simulink model "validation_model"  (R2018b)
settings: Solver=VariableStepAuto  StartTime=0.0  StopTime=10.0  RelTol=1e-3
values from neighbouring files (symbols this model uses):
  A_bike = [0 g/h_real ; 1 0]    [configuration.m]
  B_bike = [1 ; 0]    [configuration.m]
  C1_bike = a_real/(b_real*h_real)    (= 0.392543973584)    [configuration.m]
  C2_bike = 1/(b_real*h_real)    (= 1.15454109878)    [configuration.m]
  C_ini = [C1_bike*input_velocity C2_bike*input_velocity^2]    [configuration.m]
  D = zeros(3,1)    [configuration_pidTuning.m]
  delay_tf_steering = 0    [configuration.m]
  initial_states = [deg2rad(-2) deg2rad(0) deg2rad(0)]    [configuration.m]    (also in configuration_pidTuning.m)
  K_fullbike = 1    [configuration.m]
  lqr_gains = zeros(length(velocity_lqr),1+size(A_bike,1))    [lqr_design.m]
  smith_fullbike = 1    [configuration.m]
  Ts = 0.01    [configuration.m]    (also in configuration_pidTuning.m = 0.04)
  velocity_lqr = [input_velocity - 0.1 , input_velocity , input_velocity + 0.1]    [lqr_design.m]
settings Model: Creator=maximef  LastModifiedBy=maximef

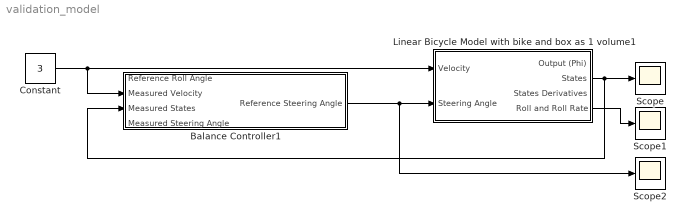
== system validation_model ==
  Balance Controller1 : Subsystem  SystemSampleTime=Ts
  Constant : Constant  Value=3
  Linear Bicycle Model with bike and box as 1 volume1 : Subsystem
  Scope : Scope
  Scope1 : Scope
  Scope2 : Scope
  wires:
  Balance Controller1/1(Reference Steering Angle) -> Scope2/1, Linear Bicycle Model with bike and box as 1 volume1/2(Steering Angle)
  Constant/1 -> Balance Controller1/2(Measured Velocity), Linear Bicycle Model with bike and box as 1 volume1/1(Velocity)
  Linear Bicycle Model with bike and box as 1 volume1/2(States) -> Scope/1, Balance Controller1/3(Measured States)
  Linear Bicycle Model with bike and box as 1 volume1/4(Roll and Roll Rate) -> Scope1/1

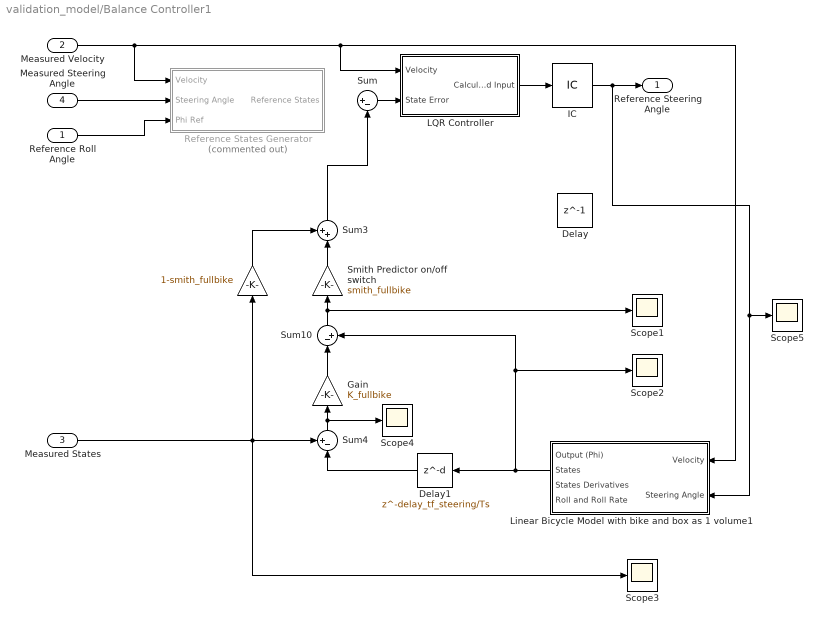
== system validation_model/Balance Controller1 ==
  Reference Roll Angle : Inport
  Measured Velocity : Inport  Port=2
  Measured States : Inport  Port=3
  Measured Steering Angle : Inport  Port=4
  " " : Gain  Gain=1-smith_fullbike
  Delay : Delay  DelayLength=1
  Delay1 : Delay  DelayLength=delay_tf_steering/Ts  SampleTime=Ts
  Gain : Gain  Gain=K_fullbike
  IC : InitialCondition  Value=0
  LQR Controller : Subsystem  TreatAsAtomicUnit=on  SystemSampleTime=Ts
  Linear Bicycle Model with bike and box as 1 volume1 : Subsystem
  Reference States Generator : Subsystem  Commented=on  SystemSampleTime=Ts
  Scope{1..5} (5 alike) : Scope
  Smith Predictor on/off switch : Gain  Gain=smith_fullbike
  Sum : Sum  Inputs=|+-
  Sum10 : Sum  Inputs=|-+
  Sum3 : Sum  Inputs=++|
  Sum4 : Sum  Inputs=+-|
  Reference Steering Angle : Outport
  wires:
  Sum/1 -> LQR Controller/2(State Error)
  LQR Controller/1(Calculated Input) -> IC/1
  Measured Velocity/1 -> Linear Bicycle Model with bike and box as 1 volume1/1(Velocity), LQR Controller/1(Velocity), Reference States Generator/1(Velocity)
  Reference Roll Angle/1 -> Reference States Generator/3(Phi Ref)
  Measured Steering Angle/1 -> Reference States Generator/2(Steering Angle)
  Measured States/1 -> " "/1, Scope3/1, Sum4/1
  " "/1 -> Sum3/1
  Sum3/1 -> Sum/2
  Linear Bicycle Model with bike and box as 1 volume1/2(States) -> Sum10/2, Scope2/1, Delay1/1
  Gain/1 -> Sum10/1
  Delay1/1 -> Sum4/2
  Smith Predictor on/off switch/1 -> Sum3/2
  Sum10/1 -> Scope1/1, Smith Predictor on/off switch/1
  Sum4/1 -> Scope4/1, Gain/1
  IC/1 -> Linear Bicycle Model with bike and box as 1 volume1/2(Steering Angle), Scope5/1, Reference Steering Angle/1

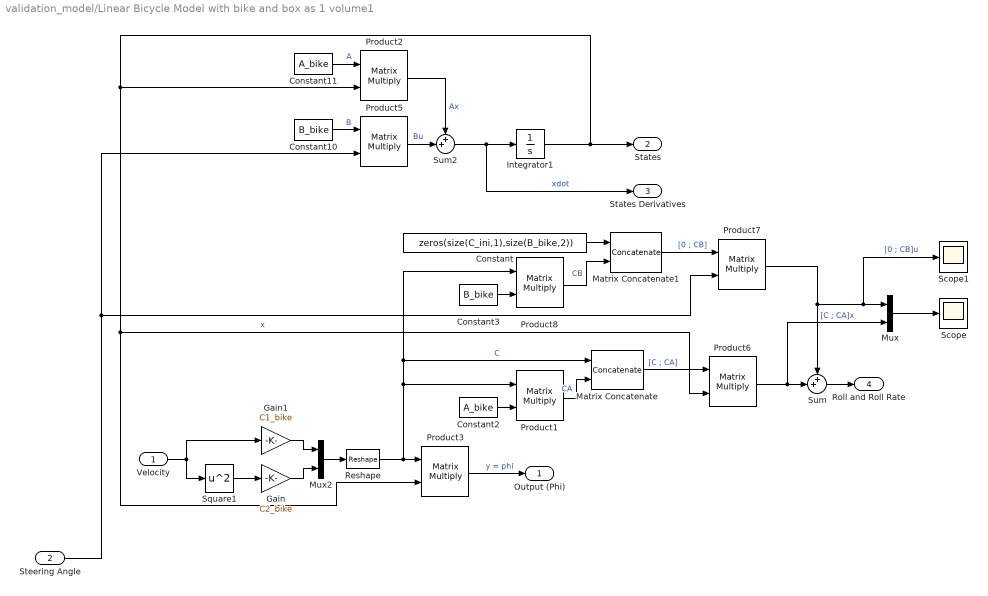
== system validation_model/Linear Bicycle Model with bike and box as 1 volume1 ==
  Velocity : Inport
  Steering Angle : Inport  Port=2
  Constant : Constant  Value=zeros(size(C_ini,1),size(B_bike,2))
  Constant10 : Constant  Value=B_bike
  Constant11 : Constant  Value=A_bike
  Constant2 : Constant  Value=A_bike
  Constant3 : Constant  Value=B_bike
  Gain : Gain  Gain=C2_bike
  Gain1 : Gain  Gain=C1_bike
  Integrator1 : Integrator  InitialCondition=[C_ini ; C_ini*A_bike]\[initial_states(1) ; initial_states(3)]
  Matrix Concatenate : Concatenate  Mode=Multidimensional array
  Matrix Concatenate1 : Concatenate  Mode=Multidimensional array
  Mux : Mux  Inputs=2
  Mux2 : Mux  Inputs=2
  Product{1..3,5..8} (7 alike) : Product  SCDEnableBlockLinearizationSpecification=on  Multiplication=Matrix(*)
  Reshape : Reshape  OutputDimensionality=Row vector (2-D)
  Scope : Scope
  Scope1 : Scope
  Square1 : Math  Operator=square  SaturateOnIntegerOverflow=on
  Sum : Sum  Inputs=++|
  Sum2 : Sum  Inputs=++|
  Output (Phi) : Outport
  States : Outport  Port=2
  States Derivatives : Outport  Port=3
  Roll and Roll Rate : Outport  Port=4
  wires:
  Integrator1/1 -> Product2/2, Product6/2, Product3/2, States/1  "x"
  Product3/1 -> Output (Phi)/1  "y = phi"
  Steering Angle/1 -> Product5/2, Product7/2
  Product2/1 -> Sum2/1  "Ax"
  Mux2/1 -> Reshape/1
  Product5/1 -> Sum2/2  "Bu"
  Sum2/1 -> Integrator1/1, States Derivatives/1  "xdot"
  Constant11/1 -> Product2/1  "A"
  Constant10/1 -> Product5/1  "B"
  Velocity/1 -> Gain1/1, Square1/1
  Square1/1 -> Gain/1
  Reshape/1 -> Product3/1, Product8/1, Matrix Concatenate/1, Product1/1  "C"
  Gain/1 -> Mux2/2
  Gain1/1 -> Mux2/1
  Sum/1 -> Roll and Roll Rate/1
  Constant2/1 -> Product1/2
  Product1/1 -> Matrix Concatenate/2  "CA"
  Matrix Concatenate/1 -> Product6/1  "[C ; CA]"
  Product6/1 -> Mux/2, Sum/2  "[C ; CA]x"
  Product7/1 -> Scope1/1, Mux/1, Sum/1  "[0 ; CB]u"
  Matrix Concatenate1/1 -> Product7/1  "[0 ; CB]"
  Product8/1 -> Matrix Concatenate1/2  "CB"
  Constant3/1 -> Product8/2
  Constant/1 -> Matrix Concatenate1/1
  Mux/1 -> Scope/1

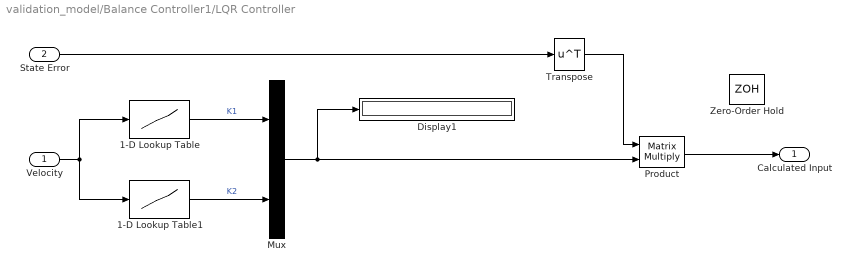
== system validation_model/Balance Controller1/LQR Controller ==
  Velocity : Inport
  State Error : Inport  Port=2
  1-D Lookup Table : Lookup_n-D  NumberOfTableDimensions=1  BreakpointsForDimension1=velocity_lqr  BreakpointsForDimension2=velocity_lqr  BreakpointsForDimension3=velocity_lqr  BreakpointsForDimension4=velocity_lqr  Table=lqr_gains(:,2)  InternalRulePriority=Speed  RndMeth=Simplest  InputSameDT=on
  1-D Lookup Table1 : Lookup_n-D  NumberOfTableDimensions=1  BreakpointsForDimension1=velocity_lqr  BreakpointsForDimension2=velocity_lqr  BreakpointsForDimension3=velocity_lqr  BreakpointsForDimension4=velocity_lqr  Table=lqr_gains(:,3)  InternalRulePriority=Speed  RndMeth=Simplest  InputSameDT=on
  Display1 : Display
  Mux : Mux  Inputs=2
  Product : Product  Multiplication=Matrix(*)
  Transpose : Math  Operator=transpose  SaturateOnIntegerOverflow=on
  Zero-Order Hold : ZeroOrderHold  SampleTime=Ts
  Calculated Input : Outport
  wires:
  1-D Lookup Table/1 -> Mux/1  "K1"
  1-D Lookup Table1/1 -> Mux/2  "K2"
  Velocity/1 -> 1-D Lookup Table1/1, 1-D Lookup Table/1
  Mux/1 -> Product/2, Display1/1
  Transpose/1 -> Product/1
  Product/1 -> Calculated Input/1
  State Error/1 -> Transpose/1

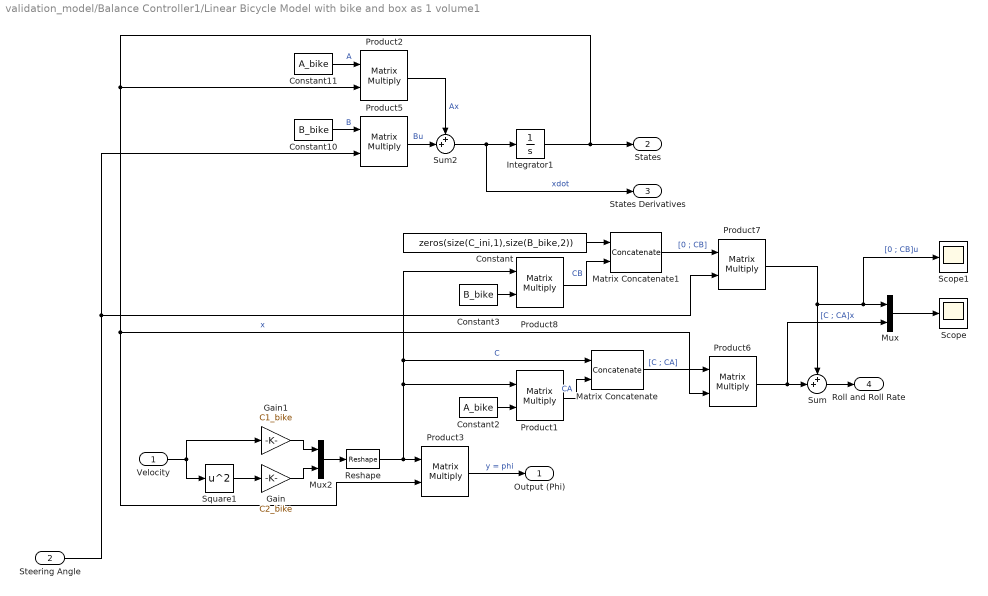
== system validation_model/Balance Controller1/Linear Bicycle Model with bike and box as 1 volume1 ==
  Velocity : Inport
  Steering Angle : Inport  Port=2
  Constant : Constant  Value=zeros(size(C_ini,1),size(B_bike,2))
  Constant10 : Constant  Value=B_bike
  Constant11 : Constant  Value=A_bike
  Constant2 : Constant  Value=A_bike
  Constant3 : Constant  Value=B_bike
  Gain : Gain  Gain=C2_bike
  Gain1 : Gain  Gain=C1_bike
  Integrator1 : Integrator  InitialCondition=[C_ini ; C_ini*A_bike]\[initial_states(1) ; initial_states(3)]
  Matrix Concatenate : Concatenate  Mode=Multidimensional array
  Matrix Concatenate1 : Concatenate  Mode=Multidimensional array
  Mux : Mux  Inputs=2
  Mux2 : Mux  Inputs=2
  Product{1..3,5..8} (7 alike) : Product  SCDEnableBlockLinearizationSpecification=on  Multiplication=Matrix(*)
  Reshape : Reshape  OutputDimensionality=Row vector (2-D)
  Scope : Scope
  Scope1 : Scope
  Square1 : Math  Operator=square  SaturateOnIntegerOverflow=on
  Sum : Sum  Inputs=++|
  Sum2 : Sum  Inputs=++|
  Output (Phi) : Outport
  States : Outport  Port=2
  States Derivatives : Outport  Port=3
  Roll and Roll Rate : Outport  Port=4
  wires:
  Integrator1/1 -> Product2/2, Product6/2, Product3/2, States/1  "x"
  Product3/1 -> Output (Phi)/1  "y = phi"
  Steering Angle/1 -> Product5/2, Product7/2
  Product2/1 -> Sum2/1  "Ax"
  Mux2/1 -> Reshape/1
  Product5/1 -> Sum2/2  "Bu"
  Sum2/1 -> Integrator1/1, States Derivatives/1  "xdot"
  Constant11/1 -> Product2/1  "A"
  Constant10/1 -> Product5/1  "B"
  Velocity/1 -> Gain1/1, Square1/1
  Square1/1 -> Gain/1
  Reshape/1 -> Product3/1, Product8/1, Matrix Concatenate/1, Product1/1  "C"
  Gain/1 -> Mux2/2
  Gain1/1 -> Mux2/1
  Sum/1 -> Roll and Roll Rate/1
  Constant2/1 -> Product1/2
  Product1/1 -> Matrix Concatenate/2  "CA"
  Matrix Concatenate/1 -> Product6/1  "[C ; CA]"
  Product6/1 -> Mux/2, Sum/2  "[C ; CA]x"
  Product7/1 -> Scope1/1, Mux/1, Sum/1  "[0 ; CB]u"
  Matrix Concatenate1/1 -> Product7/1  "[0 ; CB]"
  Product8/1 -> Matrix Concatenate1/2  "CB"
  Constant3/1 -> Product8/2
  Constant/1 -> Matrix Concatenate1/1
  Mux/1 -> Scope/1

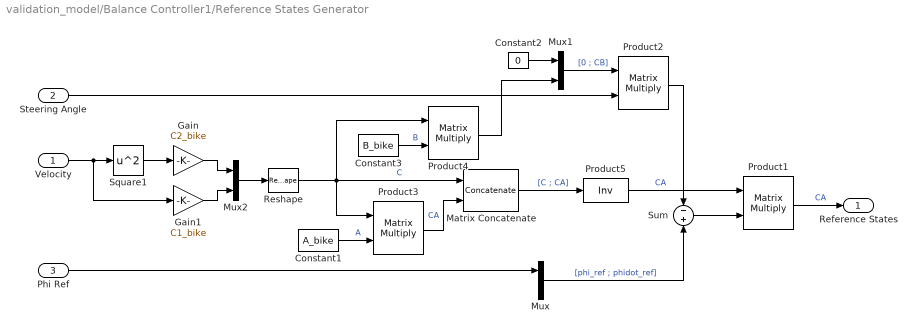
== system validation_model/Balance Controller1/Reference States Generator ==
  Velocity : Inport
  Steering Angle : Inport  Port=2
  Phi Ref : Inport  Port=3
  Constant1 : Constant  Value=A_bike
  Constant2 : Constant  Value=0
  Constant3 : Constant  Value=B_bike
  Gain : Gain  Gain=C2_bike
  Gain1 : Gain  Gain=C1_bike
  Matrix Concatenate : Concatenate  Mode=Multidimensional array
  Mux : Mux  Inputs=2
  Mux1 : Mux  Inputs=2
  Mux2 : Mux  Inputs=2
  Product{1..4} (4 alike) : Product  SCDEnableBlockLinearizationSpecification=on  Multiplication=Matrix(*)
  Product5 : Product  SCDEnableBlockLinearizationSpecification=on  Inputs=/  Multiplication=Matrix(*)
  Reshape : Reshape  OutputDimensionality=Row vector (2-D)
  Square1 : Math  Operator=square  SaturateOnIntegerOverflow=on
  Sum : Sum  Inputs=-+
  Reference States : Outport
  wires:
  Velocity/1 -> Gain1/1, Square1/1
  Gain1/1 -> Mux2/2
  Gain/1 -> Mux2/1
  Square1/1 -> Gain/1
  Reshape/1 -> Product4/1, Matrix Concatenate/1, Product3/1  "C"
  Mux2/1 -> Reshape/1
  Constant1/1 -> Product3/2  "A"
  Product3/1 -> Matrix Concatenate/2  "CA"
  Matrix Concatenate/1 -> Product5/1  "[C ; CA]"
  Mux/1 -> Sum/2  "[phi_ref ; phidot_ref]"
  Phi Ref/1 -> Mux/1
  Product2/1 -> Sum/1
  Steering Angle/1 -> Product2/2
  Mux1/1 -> Product2/1  "[0 ; CB]"
  Constant2/1 -> Mux1/1
  Product4/1 -> Mux1/2
  Constant3/1 -> Product4/2  "B"
  Sum/1 -> Product1/2
  Product1/1 -> Reference States/1  "CA"
  Product5/1 -> Product1/1  "CA"
